simulink library "constXYZT_cl"  (R2018b)
settings: Solver=VariableStepAuto  StartTime=0.0  StopTime=10.0  RelTol=1e-3
settings Model: Creator=mcobb  LastModifiedBy=mcobb

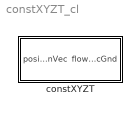
== system constXYZT_cl ==
  constXYZT : Subsystem  mask{constXYZT=0}
      mask prompts: constXYZT "env.constXYZT Object"

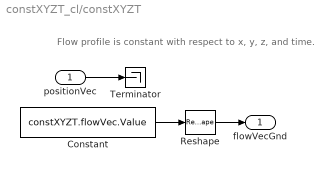
== system constXYZT_cl/constXYZT ==
  note: Flow profile is constant with respect to x, y, z, and time.
  positionVec : Inport
  Constant : Constant  Value=constXYZT.flowVec.Value
  Reshape : Reshape  OutputDimensionality=Column vector (2-D)
  Terminator : Terminator
  flowVecGnd : Outport
  wires:
  positionVec/1 -> Terminator/1
  Constant/1 -> Reshape/1
  Reshape/1 -> flowVecGnd/1
